simulink model "Multilevel5"  (R2016a)
settings: Solver=VariableStepAuto  StartTime=0.0  StopTime=0.8  RelTol=1e-3
libraries: powerlib x24
settings Model: Creator=SHIVANYA SALES  LastModifiedBy=VIP

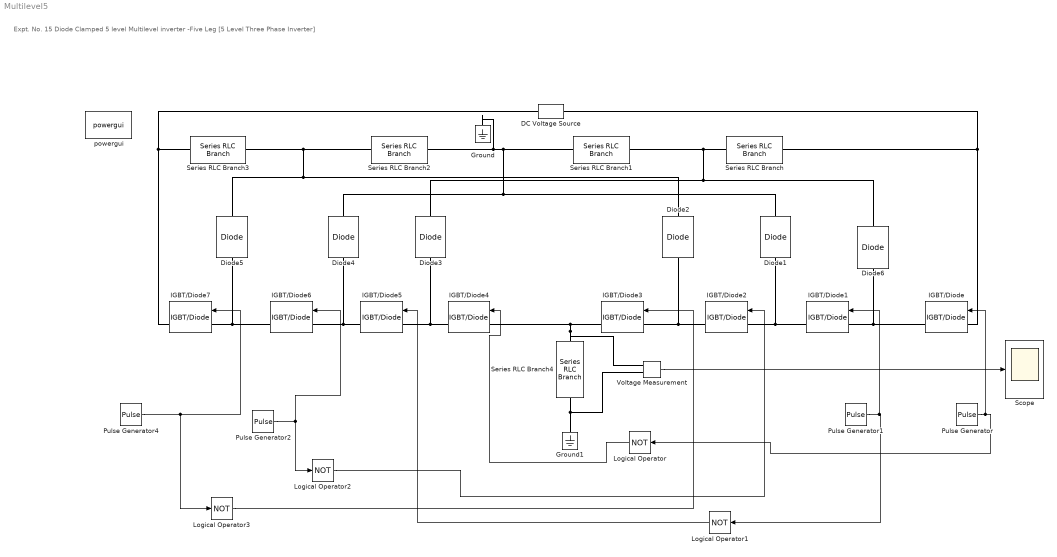
== system Multilevel5 ==
  note: Expt. No. 15 Diode Clamped 5 level Multilevel inverter -Five Leg [5 Level Three Phase Inverter]
  DC Voltage Source : powerlib/Electrical Sources/DC Voltage Source  Amplitude=50  Measurements=None
  Diode{1..6} (6 alike) : powerlib/Power Electronics/Diode  Ron=0.001  Lon=0  Vf=0.8  IC=0  UseSnubber=off  Rs=500  Cs=250e-9  Measurements=off
  Ground : powerlib/Elements/Ground  LConnTagsString=a
  Ground1 : powerlib/Elements/Ground  LConnTagsString=a
  IGBT/Diode{,1..7} (8 alike) : powerlib/Power Electronics/IGBT//Diode  Ron=1e-3  Rs=1e5  Cs=inf  Measurements=on
  Logical Operator{,1..3} (4 alike) : Logic  Operator=NOT  IconShape=distinctive  AllPortsSameDT=off  OutDataTypeStr=boolean
  Pulse Generator : DiscretePulseGenerator  PulseType=Time based  Period=0.02  PulseWidth=10  PhaseDelay=0.004
  Pulse Generator1 : DiscretePulseGenerator  PulseType=Time based  Period=0.02  PulseWidth=30  PhaseDelay=0.002
  Pulse Generator2 : DiscretePulseGenerator  PulseType=Time based  Period=0.02  PulseWidth=30  PhaseDelay=0.012
  Pulse Generator4 : DiscretePulseGenerator  PulseType=Time based  Period=0.02  PulseWidth=10  PhaseDelay=0.014
  Scope : Scope
  Series RLC Branch : powerlib/Elements/Series RLC Branch  LConnTagsString=__new0  RConnTagsString=__new0  BranchType=RC  Resistance=0.02  Inductance=1e-3  SetiL0=off  InitialCurrent=0  Capacitance=4.7e-3  Setx0=off  InitialVoltage=0  Measurements=Branch voltage and current
  Series RLC Branch1 : powerlib/Elements/Series RLC Branch  LConnTagsString=__new0  RConnTagsString=__new0  BranchType=RC  Resistance=0.02  Inductance=1e-3  SetiL0=off  InitialCurrent=0  Capacitance=4.7e-3  Setx0=off  InitialVoltage=0  Measurements=None
  Series RLC Branch2 : powerlib/Elements/Series RLC Branch  LConnTagsString=__new0  RConnTagsString=__new0  BranchType=RC  Resistance=0.02  Inductance=1e-3  SetiL0=off  InitialCurrent=0  Capacitance=4.7e-3  Setx0=off  InitialVoltage=0  Measurements=None
  Series RLC Branch3 : powerlib/Elements/Series RLC Branch  LConnTagsString=__new0  RConnTagsString=__new0  BranchType=RC  Resistance=0.02  Inductance=1e-3  SetiL0=off  InitialCurrent=0  Capacitance=4.7e-3  Setx0=off  InitialVoltage=0  Measurements=None
  Series RLC Branch4 : powerlib/Elements/Series RLC Branch  LConnTagsString=__new0  RConnTagsString=__new0  BranchType=R  Resistance=10  Inductance=1e-3  SetiL0=off  InitialCurrent=0  Capacitance=1e-6  Setx0=off  InitialVoltage=0  Measurements=None
  Voltage Measurement : powerlib/Measurements/Voltage Measurement  PhasorSimulation=off  OutputType=Complex  PSBequivalent=0
  powergui : powerlib/powergui  Priority=1  SimulationMode=Continuous  SolverType=Tustin/Backward Euler (TBE)  SampleTime=50e-6  frequency=60  SPID=off  DisableSnubberDevices=off  DisableRonSwitches=off  DisableVfSwitches=off  SwTol=0  DisplayEquations=off  Interpol=off  ExternalGateDelay=off  methode=off  Ts=10  FunctionMessages=off  echomessages=off  HookPort=off  EnableUseOfTLC=off  x0status=blocks  frequencyindice=0  Pbase=100e6  ErrMax=1e-4  Iterations=50  UnitsV=kV  UnitsW=MW  buscounter=0  RestoreLinks=warning  ResistiveCurrentMeasurement=off  Frange=[0:2:500]  Ylog=off  Xlog=on  ShowGrid=off  save=off  variable=ZData  structure=0  ZoomFFT=off  StartTime=0.0  cycles=1  DisplayStyle=1  fundamental=60  FreqAxis=off  MaxFrequency=1000  frequencyindicesteady=1  RmsSteady=1  display=off
  wires:
  Logical Operator3/1 -> IGBT/Diode3/1
  Pulse Generator2/1 -> Logical Operator2/1, IGBT/Diode6/1
  Logical Operator2/1 -> IGBT/Diode2/1
  Logical Operator1/1 -> IGBT/Diode5/1
  Pulse Generator1/1 -> IGBT/Diode1/1, Logical Operator1/1
  Logical Operator/1 -> IGBT/Diode4/1
  Pulse Generator/1 -> IGBT/Diode/1, Logical Operator/1
  Voltage Measurement/1 -> Scope/1
  Pulse Generator4/1 -> IGBT/Diode7/1, Logical Operator3/1
  connections:
  IGBT/Diode7/LConn1 -- Diode5/LConn1 -- IGBT/Diode6/RConn1
  IGBT/Diode6/LConn1 -- Diode4/LConn1 -- IGBT/Diode5/RConn1
  IGBT/Diode5/LConn1 -- Diode3/LConn1 -- IGBT/Diode4/RConn1
  IGBT/Diode4/LConn1 -- Voltage Measurement/LConn1 -- Series RLC Branch4/LConn1 -- IGBT/Diode3/RConn1
  IGBT/Diode3/LConn1 -- Diode2/RConn1 -- IGBT/Diode2/RConn1
  IGBT/Diode2/LConn1 -- IGBT/Diode1/RConn1 -- Diode1/RConn1
  IGBT/Diode7/RConn1 -- Series RLC Branch3/RConn1 -- DC Voltage Source/LConn1
  DC Voltage Source/RConn1 -- Series RLC Branch/LConn1 -- IGBT/Diode/LConn1
  Diode2/LConn1 -- Diode5/RConn1 -- Series RLC Branch2/RConn1 -- Series RLC Branch3/LConn1
  Diode1/LConn1 -- Diode4/RConn1 -- Ground/LConn1 -- Series RLC Branch2/LConn1 -- Series RLC Branch1/RConn1
  Series RLC Branch1/LConn1 -- Diode3/RConn1 -- Diode6/LConn1 -- Series RLC Branch/RConn1
  Ground1/LConn1 -- Voltage Measurement/LConn2 -- Series RLC Branch4/RConn1
  IGBT/Diode1/LConn1 -- IGBT/Diode/RConn1 -- Diode6/RConn1
